simulink model "Modelka_31"  (R2018b)
settings: Solver=ode45  StartTime=0.0  StopTime=10.0  RelTol=1e-3  EnableMultiTasking=on
settings Model: Creator=Никита Волк  LastModifiedBy=Никита Волк
settings DataIOCC: LimitDataPoints=on  SaveFormat=Array  SignalLoggingSaveFormat=ModelDataLogs
settings OptimizationCC: BooleanDataType=off
settings DebuggingCC: SaveWithParameterizedLinksMsg=none  UnderspecifiedInitializationDetection=Classic  MergeDetectMultiDrivingBlocksExec=none  SignalResolutionControl=TryResolveAllWithWarning  MultiTaskDSMMsg=warning  MultiTaskCondExecSysMsg=none
settings HardwareCC: TargetUnknown=on
settings ModelReferenceCC: PropagateSignalLabelsOutOfModel=off
settings GRTTargetCC: CombineOutputUpdateFcns=off  GRTInterface=on
settings ConfigComp: CovMetricSettings=dw  CovHtmlReporting=on

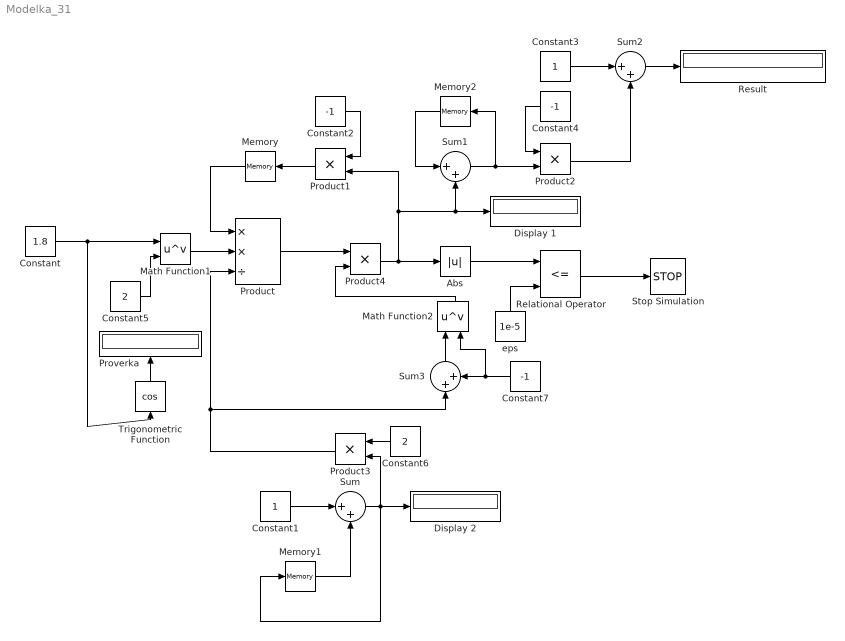
== system Modelka_31 ==
  Abs : Abs  SaturateOnIntegerOverflow=on
  Constant : Constant  Value=1.8
  Constant1 : Constant
  Constant2 : Constant  Value=-1
  Constant3 : Constant
  Constant4 : Constant  Value=-1
  Constant5 : Constant  Value=2
  Constant6 : Constant  Value=2
  Constant7 : Constant  Value=-1
  Display 1 : Display
  Display 2 : Display
  Math Function1 : Math  Operator=pow  SaturateOnIntegerOverflow=on
  Math Function2 : Math  Operator=pow  SaturateOnIntegerOverflow=on
  Memory : Memory  InitialCondition=1
  Memory1 : Memory
  Memory2 : Memory
  Product : Product  Inputs=**/  SaturateOnIntegerOverflow=on  RndMeth=Zero  InputSameDT=on  OutDataTypeStr=Inherit: Same as first input
  Product{1..4} (4 alike) : Product
  Proverka : Display
  Relational Operator : RelationalOperator  Operator=<=  RndMeth=Nearest  InputSameDT=on
  Result : Display
  Stop Simulation : Stop
  Sum{,1..3} (4 alike) : Sum  Inputs=|++  SaturateOnIntegerOverflow=on  InputSameDT=on  OutDataTypeStr=Inherit: Same as first input
  Trigonometric Function : Trigonometry  Operator=cos
  eps : Constant  Value=1e-5
  wires:
  Constant/1 -> Trigonometric Function/1, Math Function1/1
  Memory/1 -> Product/1
  Constant1/1 -> Sum/1
  Memory1/1 -> Sum/2
  Sum/1 -> Product3/2, Display 2/1, Memory1/1
  Sum1/1 -> Memory2/1, Product2/2
  Memory2/1 -> Sum1/1
  Abs/1 -> Relational Operator/1
  eps/1 -> Relational Operator/2
  Trigonometric Function/1 -> Proverka/1
  Relational Operator/1 -> Stop Simulation/1
  Constant2/1 -> Product1/1
  Product1/1 -> Memory/1
  Constant3/1 -> Sum2/1
  Constant4/1 -> Product2/1
  Product2/1 -> Sum2/2
  Sum2/1 -> Result/1
  Constant5/1 -> Math Function1/2
  Math Function1/1 -> Product/2
  Constant6/1 -> Product3/1
  Product3/1 -> Sum3/1, Product/3
  Sum3/1 -> Math Function2/1
  Constant7/1 -> Math Function2/2, Sum3/2
  Product/1 -> Product4/1
  Math Function2/1 -> Product4/2
  Product4/1 -> Abs/1, Product1/2, Display 1/1, Sum1/2
